simulink model "book1_6"  (R2020b)
settings: Solver=VariableStepAuto  StartTime=0.0  StopTime=10.0  RelTol=1e-3
settings Model: Creator=10911  LastModifiedBy=10911

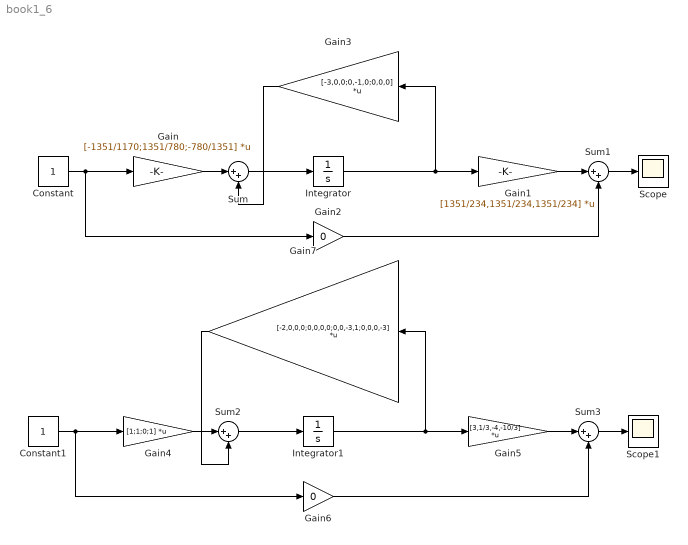
== system book1_6 ==
  Constant : Constant
  Constant1 : Constant
  Gain : Gain  Gain=[-1351/1170;1351/780;-780/1351]  Multiplication=Matrix(K*u)
  Gain1 : Gain  Gain=[1351/234,1351/234,1351/234]  Multiplication=Matrix(K*u)
  Gain2 : Gain  Gain=0
  Gain3 : Gain  Gain=[-3,0,0;0,-1,0;0,0,0]  Multiplication=Matrix(K*u)
  Gain4 : Gain  Gain=[1;1;0;1]  Multiplication=Matrix(K*u)
  Gain5 : Gain  Gain=[3,1/3,-4,-10/3]  Multiplication=Matrix(K*u)
  Gain6 : Gain  Gain=0
  Gain7 : Gain  Gain=[-2,0,0,0;0,0,0,0;0,0,-3,1;0,0,0,-3]  Multiplication=Matrix(K*u)
  Integrator : Integrator
  Integrator1 : Integrator
  Scope : Scope
  Scope1 : Scope
  Sum{,1..3} (4 alike) : Sum  Inputs=|++
  wires:
  Constant/1 -> Gain2/1, Gain/1
  Gain/1 -> Sum/1
  Sum1/1 -> Scope/1
  Integrator/1 -> Gain3/1, Gain1/1
  Gain3/1 -> Sum/2
  Sum/1 -> Integrator/1
  Gain2/1 -> Sum1/2
  Gain1/1 -> Sum1/1
  Gain5/1 -> Sum3/1
  Gain6/1 -> Sum3/2
  Sum2/1 -> Integrator1/1
  Integrator1/1 -> Gain7/1, Gain5/1
  Sum3/1 -> Scope1/1
  Constant1/1 -> Gain6/1, Gain4/1
  Gain4/1 -> Sum2/1
  Gain7/1 -> Sum2/2
